simulink model "OOK_simulink"  (R2024a)
settings: Solver=VariableStepAuto  StartTime=0.0  StopTime=20  RelTol=1e-3
libraries: dspfdesign x2
settings Model: Creator=kuria  LastModifiedBy=vaibh
settings OptimizationCC: ReuseModelBlockBuffer=off
settings RTWCC: GPUComputeCapability=3.5

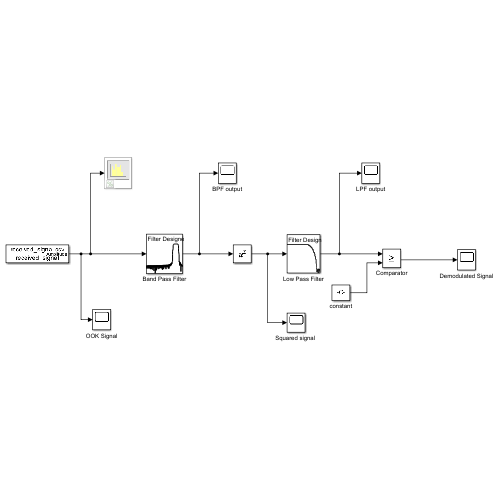
[thumbnail: Simulink's stored preview of the top-level diagram]
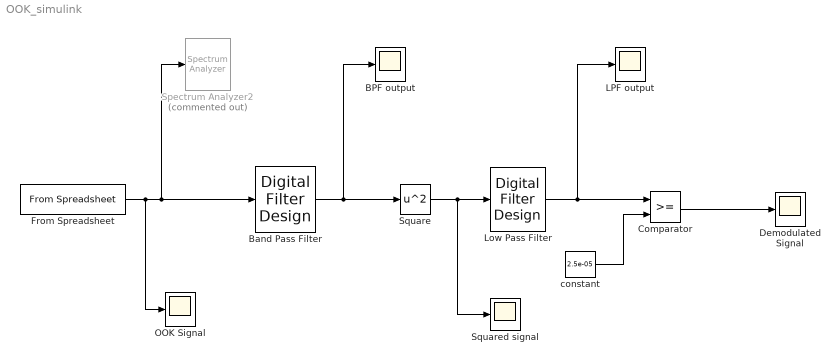
== system OOK_simulink ==
  BPF output : Scope
  Band Pass Filter : dspfdesign/Digital Filter Design  mwdsp_browser_bugfix_var=off
  Comparator : RelationalOperator  OutDataTypeStr=boolean  RndMeth=Simplest  InputSameDT=off
  Demodulated Signal : Scope
  From Spreadsheet : FromSpreadsheet  FileName=received_signal.csv  SheetName=received_signal  SampleTime=2.27e-05
  LPF output : Scope
  Low Pass Filter : dspfdesign/Digital Filter Design  mwdsp_browser_bugfix_var=off
  OOK Signal : Scope
  Spectrum Analyzer2 : SpectrumAnalyzer  Commented=on  WindowPosition=[778 434 800 450]  SpectrumType=RMS  SampleRate=1000  Span=100  StartFrequency=-500  StopFrequency=500  AveragingMethod=Exponential  SpectrumUnits=Vrms  YLimits=[-0.028839255716224546089,0.25978032093206038233]  AllowFFTLengthLessThanSamplesPerUpdate=on
  Square : Math  Operator=square
  "Squared signal " : Scope
  constant : Constant  Value=2.5e-05
  wires:
  From Spreadsheet/1 -> Band Pass Filter/1, Spectrum Analyzer2/1, OOK Signal/1
  Low Pass Filter/1 -> Comparator/1, LPF output/1
  constant/1 -> Comparator/2
  Comparator/1 -> Demodulated Signal/1
  Square/1 -> "Squared signal "/1, Low Pass Filter/1
  Band Pass Filter/1 -> Square/1, BPF output/1
